simulink model "state_space"  (R2019b)
settings: Solver=VariableStepAuto  StartTime=0.0  StopTime=10.0  RelTol=1e-3
values from neighbouring files (symbols this model uses):
  A = [Tp0-Twew0 Tzew0-Twew0;Twew0-Tp0 a*(Tzew0-Tp0)]    [WyznaczenieStatycznych.m]    (also in Wyznaczenie_K.m = [TpN-TwewN TzewN-TwewN;TwewN-TpN a*(TzewN-TpN)]; onlyfp.m = [TpN-TwewN TzewN-TwewN;TwewN-TpN a*(TzewN-TpN)]; state.m = [((-1)/Cvw)*(cp*ro_p*fpN+K1+Kw), (1/Cvw)*K1;(1/Cvp)*K1, ((-1; transmitancja.m = [TpN-TwewN TzewN-TwewN;TwewN-TpN a*(TzewN-TpN)])
  B = [(-1)*cp*ro_p*fp0*(Tz0-Twew0);0]    [WyznaczenieStatycznych.m]    (also in Wyznaczenie_K.m = [(-1)*cp*ro_p*fpN*(TzN-TwewN);0]; onlyfp.m = [(-1)*cp*ro_p*fpN*(TzN-TwewN);0]; state.m = [cp*ro_p*fpN/Cvw, Kw/Cvw;0, Kp/Cvp]; transmitancja.m = [(-1)*cp*ro_p*fpN*(TzN-TwewN);0])
  C = [cp*ro_p*fp0+K1+Kw  K1*(-1);K1*(-1) K1+Kp]    [Wyznaczenie_K.m]    (also in onlyfp.m; state.m = [1, 0;0, 1]; transmitancja.m = [cp*ro_p*fpN+K1+Kw  K1*(-1);K1*(-1) K1+Kp])
  D = [cp*ro_p*fp0*Tz0+Kw*Tzew0;Kp*Tzew0]    [Wyznaczenie_K.m]    (also in onlyfp.m; state.m = [0, 0;0, 0]; transmitancja.m = [cp*ro_p*fpN*Tz0+Kw*Tzew0;Kp*Tzew0])
  d_Tz = 0    [WyznaczenieStatycznych.m]    (also in Wyznaczenie_K.m; onlyfp.m; state.m; transmitancja.m)
  d_Tzew = 0    [WyznaczenieStatycznych.m]    (also in Wyznaczenie_K.m; onlyfp.m; state.m = 3; transmitancja.m = 3)
  t_skok = 100    [WyznaczenieStatycznych.m]    (also in Wyznaczenie_K.m = 500; onlyfp.m = 500; state.m = 500; transmitancja.m = 500)
  Tz0 = TzN    (= 30)    [WyznaczenieStatycznych.m]    (also in Wyznaczenie_K.m = vTz0(i); onlyfp.m = vTz0(i); state.m = vTz0(i); transmitancja.m = vTz0(i))
  Tzew0 = TzewN    (= -2)    [WyznaczenieStatycznych.m]    (also in Wyznaczenie_K.m = vTzew0(i); onlyfp.m = vTzew0(i); state.m = vTzew0(i); transmitancja.m = vTzew0(i))
  X0 = [Twew0,Tp0]    [state.m]
settings Model: Creator=Mariusz  LastModifiedBy=Mariusz

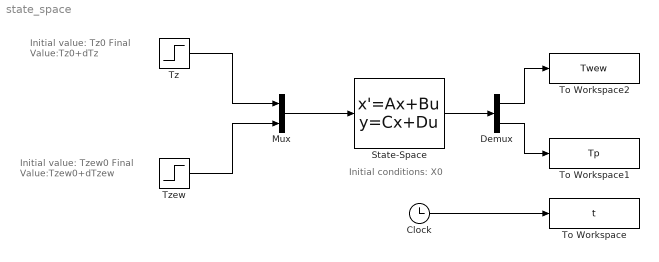
== system state_space ==
  note: Initial value: Tz0
      | Final Value:Tz0+dTz
  note: Initial conditions: X0
  note: Initial value: Tzew0
      | Final Value:Tzew0+dTzew
  Clock : Clock
  Demux : Demux  Outputs=2
  Mux : Mux  Inputs=2
  State-Space : StateSpace  A=A  B=B  C=C  D=D  InitialCondition=X0
  To Workspace : ToWorkspace  VariableName=t  SampleTime=-1
  To Workspace1 : ToWorkspace  VariableName=Tp  SampleTime=-1
  To Workspace2 : ToWorkspace  VariableName=Twew  SampleTime=-1
  Tz : Step  Time=t_skok  Before=Tz0  After=Tz0 + d_Tz  SampleTime=0
  Tzew : Step  Time=t_skok  Before=Tzew0  After=Tzew0 + d_Tzew  SampleTime=0
  wires:
  Mux/1 -> State-Space/1
  Tzew/1 -> Mux/2
  Demux/2 -> To Workspace1/1
  State-Space/1 -> Demux/1
  Clock/1 -> To Workspace/1
  Tz/1 -> Mux/1
  Demux/1 -> To Workspace2/1
